simulink library "platooning_custom_blocks"  (R2018b)
settings: Solver=VariableStepAuto  StartTime=0.0  StopTime=10.0  RelTol=1e-3
undefined symbols (not defined in the file): AccPdl_pdlbpt, AccPdl_spdbpt, AccPdl_trqMap, adj_motEffMap, BETModel, BrkPdl_brkTrq, BrkPdl_pdlbpt, Cd_Map, Cd_Map_T2, CT_accPdl_pdlbpt, CT_accPdl_spdbpt, CT_accPdl_trqMap, CT_brkPdl_brkTrq, CT_brkPdl_pdlbpt, CTModel, d_11, d_22, DiscIntNeverNeededParam, init_veh_spd_mps, max_Cd_frac, min_Cd_frac, motSpdVec, motTrqVec, msk_init_pos_m, msk_mot_cont_trq, msk_mot_num, msk_mot_spd_bpt, N_OptResults, sim_t_step, simDrv, SPHETModel, t_step
libraries: simulink x19, $bdroot x16, dspstat3 x2, custom_func x1
(part 5 of 5)

== matlab function platooning_custom_blocks/Series Parallel Hybrid Electric Truck/Series Parallel Hybrid Electric Post-Processing/Short Term Averaging Function1 ==
  data: Batt_SOC_frac input; Batt_Max_Energy input; Fuel_Used_L input; STAvg_Wh_m output; Fuel_LHV_kWhpL input; Dist_Traveled input; Dist_Window input; STAvg_L_100km output
function [STAvg_Wh_m, STAvg_L_100km] = fcn(Batt_SOC_frac, Batt_Max_Energy, Fuel_Used_L, Fuel_LHV_kWhpL, Dist_Traveled, Dist_Window)
% This function does a short term average based on the distance window for
% overall energy consumption.

% Renaming input variables to shorter names
soc = Batt_SOC_frac;
Ebatt = Batt_Max_Energy;
fuel = Fuel_Used_L;
FE = Fuel_LHV_kWhpL;
disttrvld = Dist_Traveled;
distwin = Dist_Window;

% Declaring persistent vector that stores the fuel left values - like a queue
persistent q_fuel q_soc
if isempty(q_fuel) && isempty(q_soc)
    q_fuel = fuel;
    q_soc = soc;
end

% While distance travelled is less than the distance window - fill up the
% queue

if disttrvld == 0
    STAvg_Wh_m = 0.1;
    STAvg_L_100km = 0.1;
else
    if disttrvld <= distwin
        q_fuel = [q_fuel; fuel];
        q_soc = [q_soc; soc];
        STAvg_Wh_m = ((((q_fuel(end) - q_fuel(1)) * FE) * 1000) +...
            ((q_soc(1) - q_soc(end))*Ebatt))/disttrvld;
        STAvg_L_100km = 100/(disttrvld/((q_fuel(end) - q_fuel(1)) * 1000));
    else
        q_fuel = [q_fuel(2:end); fuel];
        q_soc = [q_soc(2:end); soc];
        STAvg_Wh_m = ((((q_fuel(end) - q_fuel(1)) * FE) * 1000) +...
            ((q_soc(1) - q_soc(end))*Ebatt))/distwin;
        STAvg_L_100km = 100/(disttrvld/((q_fuel(end) - q_fuel(1)) * 1000));
    end
end

end

== matlab function platooning_custom_blocks/Battery Electric Truck/Battery Electric Powertrain Power Loss Model/A123 ESS Model/OCV_Battery/OCV Function ==
  data: soc input; ocv output; current input
function ocv = fcn(soc, current)

if current < 0
    %% 0-20 Model Fit
    if (soc <= 0.2)
        ocv = 3.17*exp(0.1*soc) - 2.76*exp(-65.25*soc);
    %% 20-80 Model Fit
    elseif (soc > 0.2 && soc <= 0.8)
        ocv = 0.155*soc + 3.2;
        % ocv = 0.165*soc + 3.20; OG
    %% 80-100 Model Fit
    else
        ocv = 0.2*(soc^74.2) + 3.33;
    end
else
%% 0-20 Model Fit
    if (soc <= 0.2)
        ocv = 3.19*exp(0.098*soc) - 1.09*exp(-48.81*soc);
    %% 20-80 Model Fit
    elseif (soc > 0.2 && soc <= 0.8)
        ocv = 0.148*soc + 3.2;
        % ocv = 0.148*soc + 3.222;
    %% 80-100 Model Fit
    else
        ocv = 0.336*(soc^108.2) + 3.34;
    end
end

== matlab function platooning_custom_blocks/Battery Electric Truck/Battery Electric Truck Energy Management System/Battery Electric Truck Regen Control Algorithm ==
  data: P_elec_dem input; P_mechbrk_W output; P_regen_avail input; Batt_SOC input; P_regenbrk_W output
function [P_mechbrk_W, P_regenbrk_W] = betregenctl(P_elec_dem,P_regen_avail,Batt_SOC)
% Battery Electric Truck Regen Control Algorithm - betregenctl
% Regen powers are negative values.
% Modelled like series regen with braking.
if P_elec_dem < 0
    if Batt_SOC <= 0.9
        if P_elec_dem >= P_regen_avail
            P_regenbrk_W = P_elec_dem;
            P_mechbrk_W = 0;
        else
            P_regenbrk_W = P_regen_avail;
            P_mechbrk_W = P_elec_dem - P_regen_avail;
        end
    else
        P_mechbrk_W = 0;
        P_regenbrk_W = 0;
    end
else
    P_mechbrk_W = 0;
    P_regenbrk_W = P_elec_dem;
end

end

== matlab function platooning_custom_blocks/Series Parallel Hybrid Electric Truck/Series Parallel Hybrid Electric Powertrain Power Loss Model/A123 ESS Model/OCV_Battery/OCV Function ==
  data: soc input; ocv output; current input
function ocv = fcn(soc, current)

if current < 0
    %% 0-20 Model Fit
    if (soc <= 0.2)
        ocv = 3.17*exp(0.1*soc) - 2.76*exp(-65.25*soc);
    %% 20-80 Model Fit
    elseif (soc > 0.2 && soc <= 0.8)
        ocv = 0.155*soc + 3.2;
        % ocv = 0.165*soc + 3.20; OG
    %% 80-100 Model Fit
    else
        ocv = 0.2*(soc^74.2) + 3.33;
    end
else
    %% 0-20 Model Fit
    if (soc <= 0.2)
        ocv = 3.19*exp(0.098*soc) - 1.09*exp(-48.81*soc);
    %% 20-80 Model Fit
    elseif (soc > 0.2 && soc <= 0.8)
        ocv = 0.148*soc + 3.2;
        % ocv = 0.148*soc + 3.222;
    %% 80-100 Model Fit
    else
        ocv = 0.336*(soc^108.2) + 3.34;
    end
end

== matlab function platooning_custom_blocks/Series Parallel Hybrid Electric Truck/Series Parallel Hybrid Electric Powertrain Power Loss Model/AWGN Function ==
  data: inp input; out output; snr input
function out = addnoise(inp,snr)

out = awgn(inp,snr,'measured');

== stateflow chart platooning_custom_blocks/Series Parallel Hybrid Electric Truck/Series Parallel Hybrid Electric Powertrain Power Loss Model/Battery EPO Logic/Battery EPO Constraint Logic ==
  state NoEPO
    du:
    epo_flag = 0;
  state EPO
    du:
    epo_flag = 1;
  (default) -> NoEPO
  NoEPO -> EPO : [LoadCurr < DchgCurrLim]
  EPO -> NoEPO : [LoadCurr >= DchgCurrLim]
  data: DchgCurrLim input; LoadCurr input; epo_flag output double

== matlab function platooning_custom_blocks/Series Parallel Hybrid Electric Truck/Series Parallel Hybrid Electric Powertrain Power Loss Model/Electric Drivetrain/MATLAB Function ==
  data: v_veh_mps input; v_veh_out_mps output; flag output
function [v_veh_out_mps,flag] = zerocheck(v_veh_mps)
    % Checks if the input speed is zero. 
    % If zero: sets the flag = 1, to change torque value to zero.
    % If not zero: sets the flag = 0, no change to the the torque value.
    
    if v_veh_mps == 0
        flag = 1;
        v_veh_out_mps = v_veh_mps;
    else
        flag = 0;
        v_veh_out_mps = v_veh_mps;
    end
end

== stateflow chart platooning_custom_blocks/Series Parallel Hybrid Electric Truck/Series Parallel Hybrid Electric Powertrain Power Loss Model/Electric Drivetrain/Motor Fault Injection/Logic ==
  state NoFault
    en:
    trigger = 1;
    du:
    trigger = 1;
  state Fault
    en:
    trigger = 0;
    du:
    trigger = 1;
  (default) -> NoFault
  NoFault -> Fault : [input == 1 && ...
      | choice == 1]
  data: trigger output double; input input; choice input

== matlab function platooning_custom_blocks/Battery Electric Truck/Battery Electric Post-Processing/Short Term Averaging Function ==
  data: Batt_SOC_frac input; STAvg_Wh_m output; Dist_Travelled input; Batt_Max_Energy input; Dist_Window input
function STAvg_Wh_m = fcn(Batt_SOC_frac,Dist_Travelled, Batt_Max_Energy, Dist_Window)
% This function does a short term average based on the distance window for
% overall energy consumption.

% Renaming input variables to shorter names
soc = Batt_SOC_frac;
Ebatt = Batt_Max_Energy;
disttrvld = Dist_Travelled;
distwin = Dist_Window;

% Declaring persistent vector that stores the SOC values - like a queue
persistent q_soc
if isempty(q_soc)
    q_soc = soc;
end

% While distance travelled is less than the distance window - fill up the
% queue

if disttrvld == 0
    STAvg_Wh_m = 1;
else
    if disttrvld <= distwin
        q_soc = [q_soc; soc];
        STAvg_Wh_m = ((q_soc(1) - q_soc(end))*Ebatt)/disttrvld;
    else
        q_soc = [q_soc(2:end); soc];
        STAvg_Wh_m = ((q_soc(1) - q_soc(end))*Ebatt)/distwin;
    end
end

end

== matlab function platooning_custom_blocks/Series Parallel Hybrid Electric Truck/Series Parallel Hybrid Electric Truck Energy Management System/Generator Load Calculator ==
  data: P_GEN_LIM_W input; P_BATT_LIM_W input; MODE_VAL input; P_elec_dem_W input; P_gen_dem_W output; P_regen_dem_W input
function P_gen_dem_W = genloadcalc(P_GEN_LIM_W, P_BATT_LIM_W, MODE_VAL, P_elec_dem_W, P_regen_dem_W)

pgencalc = max(P_GEN_LIM_W,P_BATT_LIM_W + P_regen_dem_W);

if MODE_VAL == 2
    P_gen_dem_W = pgencalc;
else
    P_gen_dem_W = 0;
end
end

== matlab function platooning_custom_blocks/Conventional Truck/Conventional Post-Processing/Short Term Averaging Function ==
  data: Fuel_Used_L input; STAvg_Wh_m output; Fuel_LHV_kWhpL input; Dist_Traveled input; Dist_Window input; STAvg_L_100km output
function [STAvg_Wh_m, STAvg_L_100km] = fcn(Fuel_Used_L, Fuel_LHV_kWhpL, Dist_Traveled, Dist_Window)
% This function does a short term average based on the distance window for
% overall energy consumption.

% Renaming input variables to shorter names
fuel = Fuel_Used_L;
FE = Fuel_LHV_kWhpL;
disttrvld = Dist_Traveled;
distwin = Dist_Window;

% Declaring persistent vector that stores the fuel left values - like a queue
persistent q_fuel
if isempty(q_fuel)
    q_fuel = fuel;
end

% While distance travelled is less than the distance window - fill up the
% queue

if disttrvld == 0
    STAvg_Wh_m = 0.1;
    STAvg_L_100km = 0.1;
else
    if disttrvld <= distwin
        q_fuel = [q_fuel; fuel];
        STAvg_Wh_m = (((q_fuel(end) - q_fuel(1)) * FE) * 1000)/disttrvld;
        STAvg_L_100km = 100/(disttrvld/((q_fuel(end) - q_fuel(1)) * 1000));
    else
        q_fuel = [q_fuel(2:end); fuel];
        STAvg_Wh_m = (((q_fuel(end) - q_fuel(1)) * FE) * 1000)/distwin;
        STAvg_L_100km = 100/(disttrvld/((q_fuel(end) - q_fuel(1)) * 1000));
    end
end

end

== matlab function platooning_custom_blocks/Conventional Truck Driver and Vehicle Acceleration Dynamics Model - Force Output/Gear Shift Logic ==
  data: upshift_req input; gear_cmd output; dnshift_req input; init_gear input; gear_ratio output; gear_rat_vec input
function [gear_cmd, gear_ratio] = fcn(upshift_req, dnshift_req, init_gear, gear_rat_vec)
    % Standard LUT based gear switch logic
    %% Pre-processing
    persistent prev_gear
    if isempty(prev_gear)
        prev_gear = init_gear;
    end
    temp_gear = prev_gear;                  % If no change in gear.
    len = length(gear_rat_vec);             % One-based idexing for gears
    
    %% Gear Shift Logic
    if temp_gear > 1 && temp_gear < len
        if upshift_req == 1
            temp_gear = temp_gear + 1;
        elseif dnshift_req == 1
            temp_gear = temp_gear - 1;
        end
    elseif temp_gear == 1
        if upshift_req == 1
            temp_gear = temp_gear + 1;
        end
    elseif temp_gear == len
        if dnshift_req == 1
            temp_gear = temp_gear - 1;
        end
    end
    %% Post-processing
    gear_cmd = temp_gear;
    gear_ratio = gear_rat_vec(temp_gear);
    prev_gear = temp_gear;
 
end

== matlab function platooning_custom_blocks/Optimal Gear Shift Algorithm/Minimum Function ==
  data: m_fuel_vec input; opt_gear output; prev_gear input
function opt_gear = minfnc(m_fuel_vec, prev_gear)
% This function finds the index of the minimum mass flow rate of the fuel
% and outputs that as the optimal gear selection.
% gear_val = [1;2;3;4;5;6;7;8;9;10];
% coder.varsize('m_fuel');
% m_fuel = m_fuel_vec;
persistent out_gear
if isempty(out_gear)
    out_gear = prev_gear;
end

MIN_VAL = min(m_fuel_vec);
MIN_VAL_INDEX = find(m_fuel_vec == MIN_VAL,1,'first');

if isempty(MIN_VAL_INDEX)
    opt_gear = out_gear;
else
    opt_gear = MIN_VAL_INDEX(1,1);
    out_gear = opt_gear;
end

end

== matlab function platooning_custom_blocks/Series Parallel Hybrid Electric Truck/Series Parallel Hybrid Electric Truck Energy Management System/Proposed ReOpt DP Algorithm/Optimal EC_Wh_m ==
  data: index input; element output; vector input
function element = idxLookup(index,vector)
% idxLookup is a custom function that returns element corresponding to
% index in a 1-D vector.
element = vector(index);
end

== matlab function platooning_custom_blocks/Series Parallel Hybrid Electric Truck/Series Parallel Hybrid Electric Truck Energy Management System/Proposed ReOpt DP Algorithm/Optimal HybMode Lookup ==
  data: index input; element output; vector input
function element = idxLookup(index,vector)
% idxLookup is a custom function that returns element corresponding to
% index in a 1-D vector.
element = vector(index);
end

== stateflow chart platooning_custom_blocks/SPHET Power Mode Selector ==
  state Stop
    du:
    Mode = 0;
  state Regen_Mode
    du:
    Mode = -1;
  state EV_Mode
    du:
    Mode = 1;
  state Series_Mode
    du:
    Mode = 2;
  state EngineOnly_Mode
    du:
    Mode = 4;
  state Parallel_Mode
    du:
    Mode = 3;
  (default) -> Stop
  Stop -> (junction 10) : [P_veh > 0 && v_spd > 0]
  (junction 10) -> (junction 17)
  (junction 13) -> Stop
  (junction 19) -> (junction 13)
  Regen_Mode -> Stop [order 1] : [v_spd == 0]
  Regen_Mode -> (junction 43) [order 4] : [ P_veh > P_lim && SOC > SOC_Lim]
  (junction 22) -> Regen_Mode
  (junction 43) -> (junction 45)
  EV_Mode -> (junction 22) [order 2] : [P_veh < 0 && ...
      | SOC < 0.8]
  (junction 40) -> Regen_Mode
  (junction 38) -> (junction 40)
  Regen_Mode -> (junction 49) [order 5] : [ P_veh > P_lim && SOC <= SOC_Lim]
  (junction 49) -> EngineOnly_Mode
  (junction 52) -> Regen_Mode
  Regen_Mode -> (junction 25) [order 2] : [(P_veh > 0 && P_veh <= P_lim)...
      |  && SOC > SOC_Lim]
  EngineOnly_Mode -> (junction 52) [order 1] : [P_veh < 0 && ...
      | SOC < 0.8]
  (junction 25) -> EV_Mode
  Series_Mode -> Regen_Mode [order 2] : [P_veh < 0 && ...
      | SOC < 0.8]
  Regen_Mode -> Series_Mode [order 3] : [(P_veh > 0 && P_veh <= P_lim)...
      |  && SOC <= SOC_Lim]
  EngineOnly_Mode -> Series_Mode [order 2] : [(P_veh > 0 && P_veh <= P_lim)...
      |  && SOC <= SOC_Lim]
  EV_Mode -> Series_Mode [order 3] : [(P_veh > 0 && P_veh <= P_lim)...
      |  && SOC <= SOC_Lim]
  EV_Mode -> (junction 19) [order 1] : [v_spd == 0]
  Series_Mode -> EV_Mode [order 1] : [(P_veh > 0 && P_veh <= P_lim)...
      |  && SOC > SOC_Lim]
  Series_Mode -> EngineOnly_Mode [order 3] : [ P_veh > P_lim &&...
      |  SOC <= SOC_Lim]
  (junction 17) -> EV_Mode
  (junction 35) -> EV_Mode
  EV_Mode -> (junction 32) [order 4] : [ P_veh > P_lim &&...
      |  SOC > SOC_Lim]
  (junction 57) -> EngineOnly_Mode
  EngineOnly_Mode -> (junction 60) [order 3] : [ P_veh > P_lim &&...
      |  SOC > SOC_Lim]
  Parallel_Mode -> (junction 57) [order 3] : [ P_veh > P_lim && SOC <= SOC_Lim]
  (junction 32) -> Parallel_Mode
  (junction 60) -> Parallel_Mode
  Parallel_Mode -> (junction 38) [order 2] : [P_veh < 0 && ...
      | SOC < SOC_MAX]
  (junction 45) -> Parallel_Mode
  Parallel_Mode -> (junction 35) [order 1] : [(P_veh > 0 && P_veh <= P_lim)...
      |  && SOC > SOC_Lim]
  data: v_spd input; P_veh input; P_lim input; SOC input; SOC_MAX input; SOC_Lim input; Mode output double

== matlab function platooning_custom_blocks/Series Parallel Hybrid Electric Truck/Series Parallel Hybrid Electric Truck Energy Management System/Proposed ReOpt DP Algorithm/Optimal Pgen Lookup ==
  data: index input; element output; vector input
function element = idxLookup(index,vector)
% idxLookup is a custom function that returns element corresponding to
% index in a 1-D vector.
element = vector(index);
end

== matlab function platooning_custom_blocks/V2V Communication Block/V2V Communication Delay Funtion ==
  data: sig_in input; sig_out output; T_DELAY input; T_STEP input; SNR_VALUE input
function sig_out = v2vcommdelay(sig_in,T_DELAY,T_STEP,SNR_VALUE)
delay_cycle = T_DELAY/T_STEP;
persistent q_sig q_ctr
if delay_cycle ~= 0
    if isempty(q_ctr)
        q_ctr = 1;
        q_sig = sig_in;
    end

    % Signal queue
    if q_ctr <= delay_cycle
        if q_ctr > 1
            q_sig = [q_sig; sig_in];
        end
        sig_out = NaN; 
        q_ctr = q_ctr + 1;
    else
        idx = q_ctr - delay_cycle - 1;
        sig_out = awgn(q_sig(1+idx,1),SNR_VALUE);
        q_sig = [q_sig(2+idx:end); sig_in];
        q_ctr = delay_cycle + 1;
    end
else
    sig_out = awgn(sig_in,SNR_VALUE);
end
end

== matlab function platooning_custom_blocks/Platoon Cd Map/MATLAB Function ==
  data: Cd_input input; Cd_output output; Cd_max input; Cd_min input
function Cd_output = fcn(Cd_input, Cd_max, Cd_min)
if ~isinf(Cd_input) && ~isnan(Cd_input)
    Cd_output = min(Cd_max,max(Cd_min, Cd_input));
else
    Cd_output = Cd_max;
end

== matlab function platooning_custom_blocks/Series Parallel Hybrid Electric Truck/Series Parallel Hybrid Electric Truck Energy Management System/Proposed ReOpt DP Algorithm/Optimal Pmot Lookup ==
  data: index input; element output; vector input
function element = idxLookup(index,vector)
% idxLookup is a custom function that returns element corresponding to
% index in a 1-D vector.
element = vector(index);
end

== matlab function platooning_custom_blocks/Series Parallel Hybrid Electric Truck/Series Parallel Hybrid Electric Truck Energy Management System/Proposed ReOpt DP Algorithm/Optimal SoC Lookup ==
  data: index input; element output; vector input
function element = idxLookup(index,vector)
% idxLookup is a custom function that returns element corresponding to
% index in a 1-D vector.
element = vector(index);
end

== stateflow chart platooning_custom_blocks/Series Parallel Hybrid Electric Truck/Series Parallel Hybrid Electric Truck Energy Management System/Proposed ReOpt DP Algorithm/Wait ==
  state Initialization
    en:
    Counter = 0;
    Trigger = 1;
  state InState
    du:
    Trigger = 1;
  state Wait1
  state Wait
  state OutState
    en:
    Trigger = 0;
    du:
    Trigger = 1;
    ex:
    Trigger = 1;
  (default) -> Initialization
  Initialization -> InState
  Wait1 -> InState : after(10.0,sec)
  Wait -> InState [order 1] : [ReOptReq == 0]
  InState -> Wait : [ReOptReq == 1]
  OutState -> Wait1 : [ReOptReq == 0]
  Wait -> OutState [order 2] : after(5.0,sec){Counter = Counter + 1;}
  data: ReOptReq input; Trigger output double; Counter output double

== stateflow chart platooning_custom_blocks/Series Parallel Hybrid Electric Truck/Series Parallel Hybrid Electric Truck Energy Management System/Regen Braking Algorithm ==
  note: %P_reg_W
  state NoBraking
    du:
    P_reg_W = 0;
    P_mechbrk_W = 0;
    P_batt_W = P_elec_W;
  state Braking
    state RegenDisabled
      du:
      P_reg_W = 0;
      P_mechbrk_W = P_elec_W;
      P_batt_W = 0;
    state RegenEnabled
      state LightBraking
        du:
        P_reg_W = P_elec_W;
        P_mechbrk_W = P_elec_W - P_reg_W;
        P_batt_W = P_reg_W;
      state HeavyBraking
        du:
        P_reg_W = P_motreg_max_W;
        P_mechbrk_W = P_elec_W - P_reg_W;
        P_batt_W = P_reg_W;
      (default) -> LightBraking
      LightBraking -> HeavyBraking : [P_elec_W <= ...
          | P_motreg_max_W]
      HeavyBraking -> LightBraking : [P_elec_W >= ...
          | P_motreg_max_W]
    (default) -> RegenDisabled
    RegenDisabled -> RegenEnabled : [SoC <= 0.75]
    RegenEnabled -> RegenDisabled : [SoC > 0.75]
  (default) -> NoBraking
  NoBraking -> Braking : [P_elec_W < 0]
  Braking -> NoBraking : [P_elec_W >= 0]
  data: P_elec_W input; P_motreg_max_W input; P_mechbrk_W output double; P_batt_W output double; P_reg_W local double; SoC input

== matlab function platooning_custom_blocks/Series Parallel Hybrid Electric Truck/Series Parallel Hybrid Electric Truck Energy Management System/SPHET Optimal Gear Shift Algorithm/Minimum Function ==
  data: m_fuel_vec input; opt_gear output; prev_gear input
function opt_gear = minfnc(m_fuel_vec, prev_gear)
% This function finds the index of the minimum mass flow rate of the fuel
% and outputs that as the optimal gear selection.
% gear_val = [1;2;3;4;5;6;7;8;9;10];
% coder.varsize('m_fuel');
% m_fuel = m_fuel_vec;
persistent out_gear
if isempty(out_gear)
    out_gear = prev_gear;
end

MIN_VAL = min(m_fuel_vec);
MIN_VAL_INDEX = find(m_fuel_vec == MIN_VAL,1,'first');

if isempty(MIN_VAL_INDEX)
    opt_gear = out_gear;
else
    opt_gear = MIN_VAL_INDEX(1,1);
    out_gear = opt_gear;
end

end

== stateflow chart platooning_custom_blocks/Series Parallel Hybrid Electric Truck/Series Parallel Hybrid Electric Truck Energy Management System/SPHET Power Mode Selector - DCARTDP ==
  state Stop
    du:
    Mode = 0;
    P_eng_W = 0;
    P_mot_W = 0;
    P_gen_W = 0;
  state Regen_Mode
    du:
    Mode = -1;
    P_eng_W = 0;
    P_mot_W = P_veh;
    P_gen_W = 0;
  state ElectricPropMode
    state EV_Mode
      du:
      Mode = 1;
      P_eng_W = 0;
      P_mot_W = P_veh;
      P_gen_W = 0;
    state Series_Mode
      du:
      Mode = 2;
      P_eng_W = 0;
      P_mot_W = P_veh;
      P_gen_W = P_gen_load_W;
    (default) -> EV_Mode
    EV_Mode -> (junction 83) : [extPgenW < -1000]
    (junction 83) -> Series_Mode
    (junction 86) -> EV_Mode
    Series_Mode -> (junction 86) : [extPgenW >= -1000]
  state CombinedPropMode
    state Parallel_Mode
      du:
      Mode = 3;
      P_eng_W = P_veh - P_LIM;
      P_mot_W = P_LIM;
      P_gen_W = 0;
    state EngineOnly_Mode
      du:
      Mode = 4;
      P_eng_W = P_veh;
      P_mot_W = 0;
      P_gen_W = 0;
    (default) -> Parallel_Mode
    Parallel_Mode -> (junction 103) : [extPmotW < 10000]
    (junction 103) -> EngineOnly_Mode
    (junction 106) -> Parallel_Mode
    EngineOnly_Mode -> (junction 106) : [extPmotW >= 10000]
  (junction 110) -> (junction 112)
  (junction 112) -> Regen_Mode
  CombinedPropMode -> (junction 110) [order 2] : [extHybMode == -1 ||...
      | P_veh < 0]
  (junction 116) -> (junction 118)
  Regen_Mode -> (junction 116) [order 3] : [extHybMode == 2]
  (junction 118) -> (junction 94)
  (default) -> Stop
  Regen_Mode -> Stop [order 1] : [v_spd == 0]
  Stop -> (junction 89)
  (junction 97) -> Regen_Mode
  (junction 89) -> (junction 97) [order 3] : [extHybMode == -1 ||...
      | P_veh < 0]
  (junction 89) -> (junction 91) [order 1] : [extHybMode == 1]
  (junction 89) -> (junction 94) [order 2] : [extHybMode == 2]
  ElectricPropMode -> Regen_Mode [order 2] : [extHybMode == -1 ||...
      | P_veh < 0]
  Regen_Mode -> (junction 91) [order 2] : [extHybMode == 1]
  (junction 91) -> ElectricPropMode
  (junction 94) -> CombinedPropMode
  ElectricPropMode -> CombinedPropMode [order 1] : [extHybMode == 2]
  CombinedPropMode -> ElectricPropMode [order 1] : [extHybMode == 1]
  data: extHybMode input; extPgenW input; extPmotW input; v_spd input; P_veh input; P_LIM input; Mode output double; P_eng_W output double; P_mot_W output double; P_gen_W output double; P_gen_load_W input

== stateflow chart platooning_custom_blocks/Series Parallel Hybrid Electric Truck/Series Parallel Hybrid Electric Truck Energy Management System/SPHET Power Mode Selector - Fixed ==
  state Stop
    du:
    Mode = 0;
    P_eng_W = 0;
    P_mot_W = 0;
    P_gen_W = 0;
  state Regen_Mode
    du:
    Mode = -1;
    P_eng_W = 0;
    P_mot_W = P_veh;
    P_gen_W = 0;
  state EV_Mode
    du:
    Mode = 1;
    P_eng_W = 0;
    P_mot_W = P_veh;
    P_gen_W = 0;
  state Series_Mode
    du:
    Mode = 2;
    P_eng_W = 0;
    P_mot_W = P_veh;
    P_gen_W = P_gen_load_W;
  state EngineOnly_Mode
    du:
    Mode = 4;
    P_eng_W = P_veh;
    P_mot_W = 0;
    P_gen_W = 0;
  state Parallel_Mode
    du:
    Mode = 3;
    P_eng_W = P_veh - P_LIM;
    P_mot_W = P_LIM;
    P_gen_W = 0;
  (default) -> Stop
  Stop -> (junction 10) : [P_veh > 0 && v_spd > 0]
  (junction 10) -> (junction 17)
  (junction 13) -> Stop
  (junction 19) -> (junction 13)
  Regen_Mode -> Stop [order 1] : [v_spd == 0]
  Regen_Mode -> (junction 43) [order 4] : [ P_veh > P_LIM && SOC > SOC_LIM]
  (junction 22) -> Regen_Mode
  (junction 43) -> (junction 45)
  EV_Mode -> (junction 22) [order 2] : [P_veh < 0 && ...
      | SOC < 0.8]
  (junction 40) -> Regen_Mode
  (junction 38) -> (junction 40)
  Regen_Mode -> (junction 49) [order 5] : [(P_veh > P_LIM &&...
      |  SOC <= SOC_LIM) || ...
      | SOC < SOC_MIN]
  (junction 49) -> EngineOnly_Mode
  Regen_Mode -> (junction 25) [order 2] : [(P_veh > 0 && P_veh <= P_LIM)...
      |  && SOC > SOC_LIM]
  (junction 52) -> Regen_Mode
  (junction 25) -> EV_Mode
  EngineOnly_Mode -> (junction 52) [order 1] : [P_veh < 0 && ...
      | SOC < 0.8]
  Series_Mode -> Regen_Mode [order 2] : [P_veh < 0 && ...
      | SOC < 0.8]
  Regen_Mode -> Series_Mode [order 3] : [(P_veh > 0 && P_veh <= P_LIM)...
      |  && SOC >= SOC_MIN + 0.05 &&...
      |  SOC <= SOC_LIM]
  EngineOnly_Mode -> Series_Mode [order 2] : [(P_veh > 0 && P_veh <= P_LIM)...
      |  && SOC >= SOC_MIN + 0.05 &&...
      |  SOC <= SOC_LIM]
  EV_Mode -> Series_Mode [order 3] : [(P_veh > 0 && P_veh <= P_LIM)...
      |  && SOC >= SOC_MIN + 0.05 &&...
      |  SOC <= SOC_LIM]
  EV_Mode -> (junction 19) [order 1] : [v_spd == 0]
  Series_Mode -> EngineOnly_Mode [order 3] : [(P_veh > P_LIM &&...
      |  SOC <= SOC_LIM) || ...
      | SOC < SOC_MIN]
  Series_Mode -> EV_Mode [order 1] : [(P_veh > 0 && P_veh <= P_LIM)...
      |  && SOC > SOC_LIM]
  (junction 17) -> EV_Mode
  (junction 35) -> EV_Mode
  EV_Mode -> (junction 32) [order 4] : [ P_veh > P_LIM &&...
      |  SOC > SOC_LIM]
  EV_Mode -> (junction 79) [order 5] : [(P_veh > P_LIM &&...
      |  SOC <= SOC_LIM) || ...
      | SOC < SOC_MIN]
  Parallel_Mode -> Series_Mode [order 4] : [(P_veh > 0 && P_veh <= P_LIM)...
      |  && SOC >= SOC_MIN + 0.05 &&...
      |  SOC <= SOC_LIM]
  (junction 81) -> EngineOnly_Mode
  (junction 57) -> EngineOnly_Mode
  EngineOnly_Mode -> (junction 60) [order 3] : [ P_veh > P_LIM &&...
      |  SOC > SOC_LIM]
  (junction 79) -> (junction 81)
  Parallel_Mode -> (junction 57) [order 3] : [(P_veh > P_LIM &&...
      |  SOC <= SOC_LIM) || ...
      | SOC < SOC_MIN]
  (junction 60) -> Parallel_Mode
  (junction 32) -> Parallel_Mode
  Parallel_Mode -> (junction 38) [order 2] : [P_veh < 0 && ...
      | SOC < SOC_MAX]
  (junction 45) -> Parallel_Mode
  Parallel_Mode -> (junction 35) [order 1] : [(P_veh > 0 && P_veh <= P_LIM)...
      |  && SOC > SOC_LIM]
  data: v_spd input; P_veh input; SOC input; SOC_MAX input; SOC_MIN input; P_LIM input; SOC_LIM input; Mode output double; P_eng_W output double; P_mot_W output double; P_gen_W output double; P_gen_load_W input

== matlab function platooning_custom_blocks/Battery Electric Truck/Battery Electric Powertrain Power Loss Model/AWGN Function ==
  data: inp input; out output; snr input
function out = addnoise(inp,snr)

out = awgn(inp,snr,'measured');

== stateflow chart platooning_custom_blocks/Battery Electric Truck/Battery Electric Powertrain Power Loss Model/Battery EPO Logic/Battery EPO Constraint Logic ==
  state NoEPO
    du:
    epo_flag = 0;
  state EPO
    du:
    epo_flag = 1;
  (default) -> NoEPO
  NoEPO -> EPO : [LoadCurr < DchgCurrLim]
  EPO -> NoEPO : [LoadCurr >= DchgCurrLim]
  data: DchgCurrLim input; LoadCurr input; epo_flag output double

== matlab function platooning_custom_blocks/Battery Electric Truck/Battery Electric Powertrain Power Loss Model/Electric Drivetrain/MATLAB Function ==
  data: v_veh_mps input; v_veh_out_mps output; flag output
function [v_veh_out_mps,flag] = zerocheck(v_veh_mps)
    % Checks if the input speed is zero. 
    % If zero: sets the flag = 1, to change torque value to zero.
    % If not zero: sets the flag = 0, no change to the the torque value.
    
    if v_veh_mps == 0
        flag = 1;
        v_veh_out_mps = v_veh_mps;
    else
        flag = 0;
        v_veh_out_mps = v_veh_mps;
    end
end

== stateflow chart platooning_custom_blocks/Battery Electric Truck/Battery Electric Powertrain Power Loss Model/Electric Drivetrain/Motor Fault Injection/Logic ==
  state NoFault
    en:
    trigger = 1;
    du:
    trigger = 1;
  state Fault
    en:
    trigger = 0;
    du:
    trigger = 1;
  (default) -> NoFault
  NoFault -> Fault : [input == 1 && ...
      | choice == 1]
  data: trigger output double; input input; choice input
